simulink model "HW6prob2c"  (Simulink 7.8)
settings: Solver=ode45  StartTime=0.0  StopTime=6  MaxStep=.01  RelTol=1e-3
values from neighbouring files (symbols this model uses):
  A = [0, 1; -2, -3]    [16-31-hw-6.m]
  B = [0; 1]    [16-31-hw-6.m]
  Kc = lqr(Aprime, B1prime, Qtild, Rtild)    [16-31-hw-6.m]
  uncert = 0.1    [16-31-hw-6.m]
settings Model: Creator=Dan  LastModifiedBy=Dan

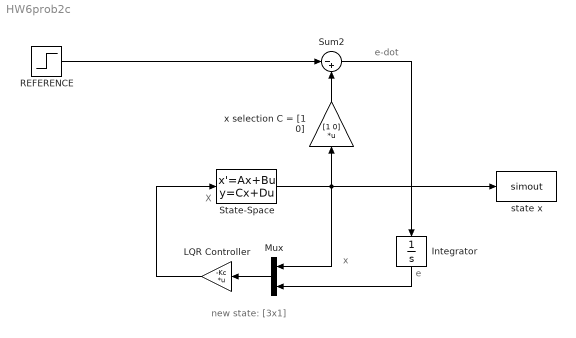
== system HW6prob2c ==
  note: X
  note: e-dot
  note: e
  note: x
  note: new state: [3x1]
  Integrator : Integrator
  LQR Controller : Gain  Gain=-Kc  Multiplication=Matrix(K*u)
  Mux : Mux  Inputs=2
  REFERENCE : Step  SampleTime=0
  State-Space : StateSpace  A=A+eye(2,2)*uncert  B=B  C=eye(2,2)  D=[0;0]
  Sum2 : Sum  Inputs=|-+
  state x : ToWorkspace  VariableName=simout  SampleTime=-1  SaveFormat=Array
  x selection C = [1 0] : Gain  Gain=[1 0]  Multiplication=Matrix(K*u)
  wires:
  x selection C = [1 0]/1 -> Sum2/2
  Sum2/1 -> Integrator/1
  Integrator/1 -> Mux/2
  LQR Controller/1 -> State-Space/1
  Mux/1 -> LQR Controller/1
  REFERENCE/1 -> Sum2/1
  State-Space/1 -> Mux/1, x selection C = [1 0]/1, state x/1
